simulink model "extkalmfilt_simdemo"  (R2020b)
settings: Solver=VariableStepAuto  StartTime=0.0  StopTime=tf  RelTol=1e-3
model workspace (MATLAB code in the model file):
  | %global Cv Ac Ts Fi_ss Qtrue
  | 
  | % Tank properties
  | Ac = 1; Cv = 3;
  | 
  | % Initial conditions
  | x0 = 1;
  | 
  | % Steady-state flow
  | Fi_ss = 3;
  | 
  | % Sampling interval
  | Ts = 0.1;
  | 
  | % Final time and time vector
  | tf = 127.4;
  | kvec = (0:Ts:tf)';
  | N = length(kvec);
  | 
  | % Input sequence (deviation from steady-state)
  | ukvec = idinput(N,'prbs',[0 0.2],[-0.05 0.05]);
  | simin = [kvec ukvec];
  | 
  | % Process and measurement noise covariances
  | Qtrue = 0.01;
  | Rtrue = 0.01;
libraries: sharedTrackingLibrary x1
settings Model: OrderedModelArguments=off  Creator=arun  LastModifiedBy=HP

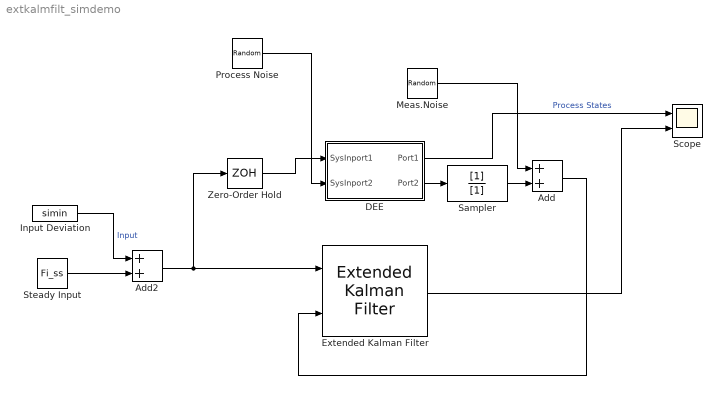
== system extkalmfilt_simdemo ==
  Add : Sum
  Add2 : Sum
  DEE : Subsystem  mask(Differential Equation Editor (DEE)){}
      settings: OpenFcn=diffeqed
      mask Display: disp('Liquid Level \n System')
  Extended Kalman Filter : sharedTrackingLibrary/Extended Kalman Filter  StateTransitionFcn=liqlstatetrans_fun_old  HasStateTransitionJacobianFcn=off  HasAdditiveProcessNoise=Additive  ProcessNoise=Qtrue  HasTimeVaryingProcessNoise=off  HasStateTransitionFcnExtraArgument=1  InitialState=1  InitialStateCovariance=0.001  MeasurementFcn1=liqlmeas_fun  HasMeasurementJacobianFcn1=off  HasMeasurementEnablePort1=off  HasAdditiveMeasurementNoise1=Additive  MeasurementNoise1=Rtrue  HasTimeVaryingMeasurementNoise1=off  HasMeasurementFcnExtraArgument1=0  MeasurementFcn2=myMeasurementFcn  HasMeasurementJacobianFcn2=off  HasMeasurementEnablePort2=off  HasAdditiveMeasurementNoise2=Additive  MeasurementNoise2=1  HasTimeVaryingMeasurementNoise2=off  HasMeasurementFcnExtraArgument2=0  MeasurementFcn3=myMeasurementFcn  HasMeasurementJacobianFcn3=off  HasMeasurementEnablePort3=off  HasAdditiveMeasurementNoise3=Additive  MeasurementNoise3=1  HasTimeVaryingMeasurementNoise3=off  HasMeasurementFcnExtraArgument3=0  MeasurementFcn4=myMeasurementFcn  HasMeasurementJacobianFcn4=off  HasMeasurementEnablePort4=off  HasAdditiveMeasurementNoise4=Additive  MeasurementNoise4=1  HasTimeVaryingMeasurementNoise4=off  HasMeasurementFcnExtraArgument4=0  MeasurementFcn5=myMeasurementFcn  HasMeasurementJacobianFcn5=off  HasMeasurementEnablePort5=off  HasAdditiveMeasurementNoise5=Additive  MeasurementNoise5=1  HasTimeVaryingMeasurementNoise5=off  HasMeasurementFcnExtraArgument5=0  EnableMultirate=off  StateTransitionFcnSampleTime=1  MeasurementFcn1SampleTime=1  MeasurementFcn2SampleTime=1  MeasurementFcn3SampleTime=1  MeasurementFcn4SampleTime=1  MeasurementFcn5SampleTime=1  UseCurrentEstimator=on  OutputStateCovariance=off  DataType=double  SampleTime=Ts  NumberOfMeasurements=1
      settings: SourceProductBaseCode=CT,DR,TF,ID,LP,NV,AR,RO,RR,UV,VE
  Input Deviation : FromWorkspace  VariableName=simin  SampleTime=Ts  Interpolate=off  OutputAfterFinalValue=Holding final value
  Meas.Noise : RandomNumber  Variance=Rtrue  Seed=4781  SampleTime=Ts
  Process Noise : RandomNumber  Variance=Qtrue  Seed=38760  SampleTime=Ts
  Sampler : DiscreteFilter  Denominator=[1]  SampleTime=Ts
  Scope : Scope  NumInputPorts=2
  Steady Input : Constant  Value=Fi_ss  SampleTime=Ts
  Zero-Order Hold : ZeroOrderHold  SampleTime=Ts
  wires:
  DEE/1(Port1) -> Scope/1  "Process States"
  Meas.Noise/1 -> Add/1
  Zero-Order Hold/1 -> DEE/1(SysInport1)
  Add/1 -> Extended Kalman Filter/2
  Extended Kalman Filter/1 -> Scope/2
  Steady Input/1 -> Add2/2
  Add2/1 -> Extended Kalman Filter/1, Zero-Order Hold/1
  Input Deviation/1 -> Add2/1  "Input"
  DEE/2(Port2) -> Sampler/1
  Sampler/1 -> Add/2
  Process Noise/1 -> DEE/2(SysInport2)

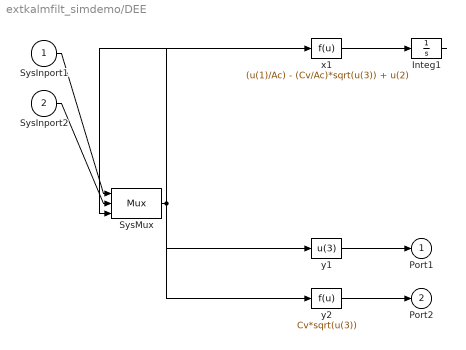
== system extkalmfilt_simdemo/DEE ==
  SysInport1 : Inport
  SysInport2 : Inport  Port=2
  Integ1 : Integrator  InitialCondition=x0
  SysMux : Mux  Inputs=3
  x1 : Fcn  Expr=(u(1)/Ac) - (Cv/Ac)*sqrt(u(3)) + u(2)
  y1 : Fcn  Expr=u(3)
  y2 : Fcn  Expr=Cv*sqrt(u(3))
  Port1 : Outport
  Port2 : Outport  Port=2
  wires:
  SysInport1/1 -> SysMux/1
  SysInport2/1 -> SysMux/2
  SysMux/1 -> x1/1, y1/1, y2/1
  x1/1 -> Integ1/1
  Integ1/1 -> SysMux/3
  y1/1 -> Port1/1
  y2/1 -> Port2/1
